simulink model "pendulum_calc"  (R2019b)
settings: Solver=VariableStepAuto  StartTime=0.0  StopTime=10.0  RelTol=1e-3
settings Model: Creator=Admin  LastModifiedBy=Admin

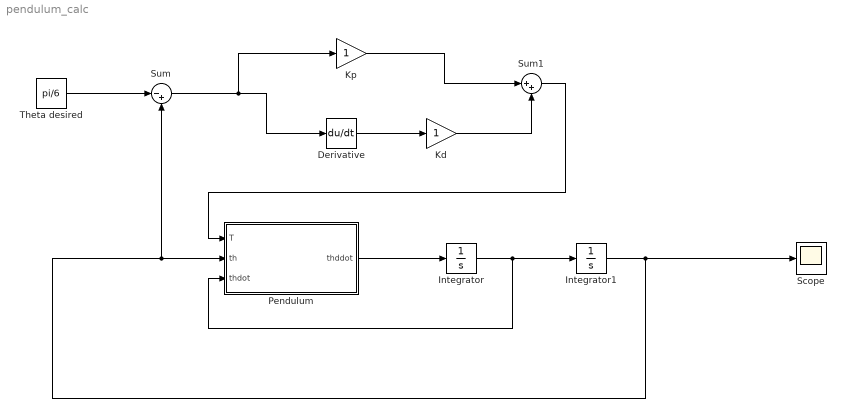
== system pendulum_calc ==
  Derivative : Derivative
  Integrator : Integrator
  Integrator1 : Integrator  InitialCondition=pi/2
  Kd : Gain
  Kp : Gain
  Pendulum : MATLAB Function  TreatAsAtomicUnit=on
  Scope : Scope
  Sum : Sum  Inputs=|-+
  Sum1 : Sum  Inputs=|++
  Theta desired : Constant  Value=pi/6
  wires:
  Pendulum/1(thddot) -> Integrator/1
  Integrator/1 -> Pendulum/3(thdot), Integrator1/1
  Theta desired/1 -> Sum/1
  Sum/1 -> Kp/1, Derivative/1
  Derivative/1 -> Kd/1
  Kp/1 -> Sum1/1
  Kd/1 -> Sum1/2
  Sum1/1 -> Pendulum/1(T)
  Integrator1/1 -> Pendulum/2(th), Sum/2, Scope/1

== matlab function pendulum_calc/Pendulum ==
  data: T input; thddot output; th input; thdot input
function thddot = pendulum_calc(T,th,thdot)

m=1;
g=9.81;
l=1;

thddot = (-T+m*g*l*sin(th))/(m*l^2);
